simulink model "rotpentemplate_cleanedup"  (R2023a)
settings: Solver=VariableStepDiscrete  StartTime=0.0  StopTime=120  RelTol=1e-3  EnableMultiTasking=on
values from neighbouring files (symbols this model uses):
  adingain = [adingain 1 1 1 1 1]    [hwinit.m]    (also in theta2_bottomswing.mat = [1.276 1.276 1 1 1 1 1])
  adinoffs = [adinoffs 0 0 0 0 0]    [hwinit.m]    (also in theta2_bottomswing.mat = [-3.773 -1.223 0 0 0 0 0])
  daoutgain = 1*[-6]    [hwinit.m]    (also in theta2_bottomswing.mat = -6)
  daoutoffs = [0.00]    [hwinit.m]    (also in theta2_bottomswing.mat = 0)
  h = 0.01    [hwinit.m]    (also in mpc_controller.m = zeros(dim.nx+dim.nu, 1); theta2_bottomswing.mat = 0.05)
  K_lqr = [K_lqr, 0, 0]    [mpc_controller.m]
  sys_dis = c2d(sys_ct, h)    [mpc_controller.m]
undefined symbols (not defined in the file or in its folder): DiscIntNeverNeededParam, Discrete, Time
libraries: simulink x3, ctrlSharedLib x1
settings Model: Creator=rbabuska  LastModifiedBy=ellyb
settings SolverCC: AlgebraicLoopSolver=TrustRegion
settings DataIOCC: LimitDataPoints=on  SaveFormat=Array  ReturnWorkspaceOutputs=off  SignalLoggingName=sigsOut
settings OptimizationCC: BooleanDataType=off  ExpressionDepthLimit=2147483647  InitFltsAndDblsToZero=on  LifeSpan=inf
settings DebuggingCC: SaveWithParameterizedLinksMsg=none  SignalResolutionControl=TryResolveAllWithWarning  MultiTaskDSMMsg=warning  MultiTaskCondExecSysMsg=none  UnconnectedInputMsg=warning  UnconnectedOutputMsg=warning  UnconnectedLineMsg=warning  AllowSymbolicDim=off  StateNameClashWarn=warning  SFUnexpectedBacktrackingDiag=warning  SFNoUnconditionalDefaultTransitionDiag=warning  SFExecutionAtInitializationDiag=none  ArithmeticOperatorsInVariantConditions=warning
settings HardwareCC: ProdBitPerPointer=32  ProdBitPerSizeT=32  ProdBitPerPtrDiffT=32  ProdLargestAtomicFloat=None  ProdIntDivRoundTo=Undefined  ProdEndianess=Unspecified  ProdWordSize=32  ProdHWDeviceType=32-bit Generic  TargetUnknown=on
settings ModelReferenceCC: EnableRefExpFcnMdlSchedulingChecks=on  PropagateSignalLabelsOutOfModel=off
settings SFSimCC: SimUseLocalCustomCode=off  CustomCodeUndefinedFunction=UseInterfaceOnly
settings RTWCC: RTWUseLocalCustomCode=off  DLArmComputeVersion=19.05
settings CodeAppCC: StateflowObjectComments=on
settings GRTTargetCC: TargetFcnLib=ansi_tfl_tmw.mat  TargetLangStandard=C89/C90 (ANSI)  CombineOutputUpdateFcns=off  GRTInterface=on
settings ConfigComp: CovMetricSettings=dw  CovSaveCumulativeToWorkspaceVar=on  CovSaveSingleToWorkspaceVar=on  CovExternalEMLEnable=off

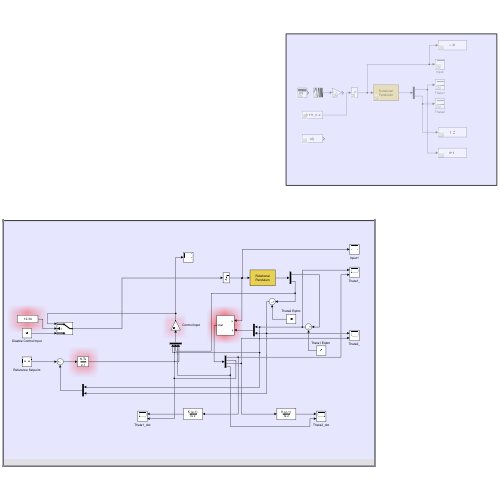
[thumbnail: Simulink's stored preview of the top-level diagram]
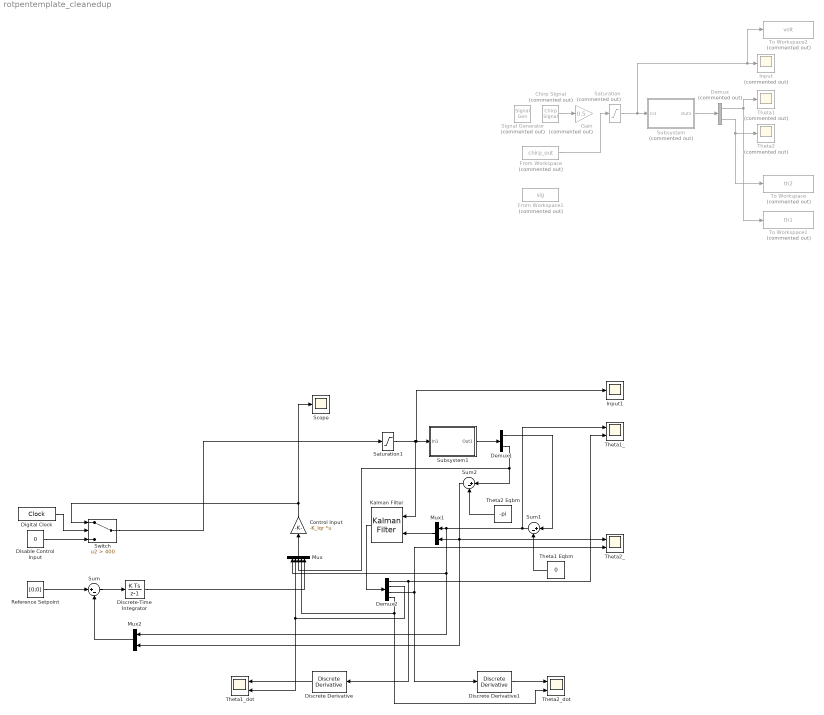
== system rotpentemplate_cleanedup ==
  Chirp Signal : simulink/Sources/Chirp Signal  Commented=on  f1=2  T=45  f2=6
  Control Input : Gain  Gain=-K_lqr  Multiplication=Matrix(K*u)
  Demux : Demux  Commented=on  Outputs=2
  Demux1 : Demux  Outputs=2
  Demux2 : Demux
  Digital Clock : DigitalClock  SampleTime=h
  Disable Control Input : Constant  Value=0  SampleTime=-1
  Discrete Derivative : simulink/Discrete/Discrete Derivative  gainval=1.0  ICPrevScaledInput=0.0  OutMin=[]  OutMax=[]  OutDataType=fixdt(1, 16)  OutScaling=2^-10  DoSatur=off
  Discrete Derivative1 : simulink/Discrete/Discrete Derivative  gainval=1.0  ICPrevScaledInput=0.0  OutMin=[]  OutMax=[]  OutDataType=fixdt(1, 16)  OutScaling=2^-10  DoSatur=off
  Discrete-Time Integrator : DiscreteIntegrator  SampleTime=h  ICPrevOutput=DiscIntNeverNeededParam  ICPrevScaledInput=DiscIntNeverNeededParam
  From Workspace : FromWorkspace  Commented=on  VariableName=chirp_out  SampleTime=h
  From Workspace1 : FromWorkspace  Commented=on  VariableName=sig  SampleTime=h
  Gain : Gain  Commented=on  Gain=0.5
  Input : Scope  Commented=on
  Input1 : Scope
  Kalman Filter : ctrlSharedLib/Kalman Filter  TimeDomain=Discrete-Time  UseCurrentEstimator=on  ModelSource=Individual A, B, C, D matrices  ModelSourceVariable=ss(0.95,1,1,0,1)  A=sys_dis.A  B=sys_dis.B  C=sys_dis.C  D=sys_dis.D  NumberOfStates=1  NumberOfInputs=1  NumberOfOutputs=1  InitialEstimateSource=Dialog  X0=0  P0=10  UseK=off  UseGH=off  NumberOfProcessNoiseInputs=1  G=1  TimeInvariantG=on  H=0  TimeInvariantH=on  Q=diag([0.1^2 0.1^2 0.01^2 0.001^2])  TimeInvariantQ=on  R=diag([0.01^2 0.05^2])  TimeInvariantR=on  N=0  TimeInvariantN=on  AddInputPort=on  AddEnablePort=off  OutputEstimatedY=off  OutputP=off  Ts=-1
  Mux : Mux  Inputs=5
  Mux1 : Mux  Inputs=2
  Mux2 : Mux  Inputs=2
  Reference Setpoint : Constant  Value=[0;0]  SampleTime=-1
  Saturation : Saturate  Commented=on  UpperLimit=1  LowerLimit=-1
  Saturation1 : Saturate  UpperLimit=1  LowerLimit=-1
  Scope : Scope
  Signal Generator : SignalGenerator  Commented=on  Amplitude=0.3*1
  Subsystem : Subsystem  Commented=on
      mask Display: disp('Rotational\nPendulum')
  Subsystem1 : Subsystem
      mask Display: disp('Rotational\nPendulum')
  Sum : Sum  Inputs=|+-
  Sum1 : Sum  Inputs=|+-
  Sum2 : Sum  Inputs=|+-
  Switch : Switch  Criteria=u2 > Threshold  Threshold=400  SaturateOnIntegerOverflow=off  InputSameDT=off
  Theta1 : Scope  Commented=on
  "Theta1 Eqbm " : Constant  Value=0  SampleTime=-1
  Theta1_ : Scope  NumInputPorts=2
  Theta1_dot : Scope  NumInputPorts=2
  Theta2 : Scope  Commented=on
  Theta2 Eqbm : Constant  Value=-pi  SampleTime=-1
  Theta2_ : Scope  NumInputPorts=2
  Theta2_dot : Scope  NumInputPorts=2
  To Workspace : ToWorkspace  Commented=on  VariableName=th2  SaveFormat=Timeseries  SampleTime=-1
  To Workspace1 : ToWorkspace  Commented=on  VariableName=th1  SaveFormat=Timeseries  SampleTime=-1
  To Workspace2 : ToWorkspace  Commented=on  VariableName=volt  SaveFormat=Timeseries  SampleTime=-1
  wires:
  Saturation/1 -> Subsystem/1(In1), To Workspace2/1, Input/1
  Subsystem/1(Out1) -> Demux/1
  Demux/1 -> To Workspace1/1, Theta1/1
  Demux/2 -> To Workspace/1, Theta2/1
  Chirp Signal/1 -> Gain/1
  From Workspace/1 -> Saturation/1
  Demux1/1 -> Sum1/1
  Demux1/2 -> Sum2/1, Mux/3
  Subsystem1/1(Out1) -> Demux1/1
  Saturation1/1 -> Subsystem1/1(In1), Input1/1, Kalman Filter/1
  Kalman Filter/1 -> Demux2/1
  Demux2/3 -> Theta2_/2, Discrete Derivative1/1
  Mux/1 -> Control Input/1
  Demux2/2 -> Theta1_dot/2, Mux/2
  Demux2/1 -> Theta1_/2, Discrete Derivative/1
  Demux2/4 -> Theta2_dot/2, Mux/4
  "Theta1 Eqbm "/1 -> Sum1/2
  Mux1/1 -> Kalman Filter/2
  Discrete Derivative1/1 -> Theta2_dot/1
  Discrete Derivative/1 -> Theta1_dot/1
  Theta2 Eqbm/1 -> Sum2/2
  Sum2/1 -> Mux1/2, Mux2/2, Theta2_/1
  Sum1/1 -> Mux2/1, Mux/1, Mux1/1, Theta1_/1
  Switch/1 -> Saturation1/1
  Control Input/1 -> Scope/1, Switch/1
  Digital Clock/1 -> Switch/2
  Disable Control Input/1 -> Switch/3
  Sum/1 -> Discrete-Time Integrator/1
  Mux2/1 -> Sum/2
  Reference Setpoint/1 -> Sum/1
  Discrete-Time Integrator/1 -> Mux/5

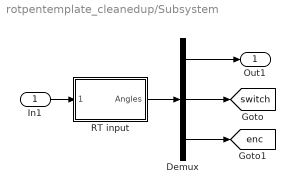
== system rotpentemplate_cleanedup/Subsystem ==
  In1 : Inport
  Demux : Demux  Outputs=[2 4 1]
  RT input : Subsystem  mask{Ts=h, channels=[6 7]}
      mask prompts: Ts "Sample time [s]:"; channels "Channels to read (e.g., [6 7])"
      mask init:
      | hwinit;
      | 
      | % initialize FPGA
      | fugihandle = fugiboard('Open', 'Pendulum1');
      | fugihandle.WatchdogTimeout = 0.5;
      | fugiboard('SetParams', fugihandle);
      | fugiboard('Write', fugihandle, 0, 0, 0, 0);  % dummy write to sync interface board
      | fugiboard('Write', fugihandle, 5, 1, 0, 0);  % reset position, activate relay
      | data = fugiboard('Read', fugihandle);        % get version info from FPGA
      | % model = bitshift(data(1), -5); 
      | % version = bitand(data(1), 31);
      | % disp(sprintf('FPGA setup %d, version %d', model, version)); % for the B&P it should say 1 1, or else there is a problem
      | fugiboard('Write', fugihandle, 0, 1, 0, 0);  % end reset
      | pause(0.1);                         % give relay some time to respond
      mask Display: disp('Rotational\nPendulum')
  Out1 : Outport
  tag scope: enc=global, switch=global
  wires:
  RT input/1(Angles) -> Demux/1
  Demux/1 -> Out1/1
  Demux/2 -> [switch]
  Demux/3 -> [enc]
  In1/1 -> RT input/1(Motors)

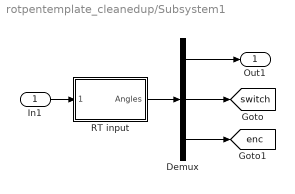
== system rotpentemplate_cleanedup/Subsystem1 ==
  In1 : Inport
  Demux : Demux  Outputs=[2 4 1]
  RT input : Subsystem  mask{Ts=h, channels=[6 7]}
      mask prompts: Ts "Sample time [s]:"; channels "Channels to read (e.g., [6 7])"
      mask init: same as rotpentemplate_cleanedup/Subsystem/RT input
      mask Display: disp('Rotational\nPendulum')
  Out1 : Outport
  tag scope: enc=global, switch=global
  wires:
  RT input/1(Angles) -> Demux/1
  Demux/1 -> Out1/1
  Demux/2 -> [switch]
  Demux/3 -> [enc]
  In1/1 -> RT input/1(Motors)

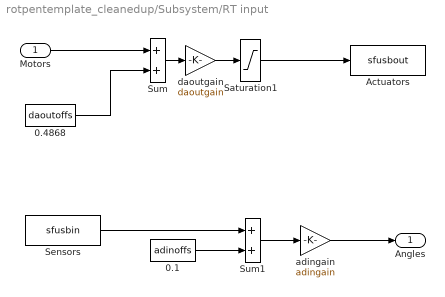
== system rotpentemplate_cleanedup/Subsystem/RT input ==
  Motors : Inport
  0.1 : Constant  Value=adinoffs
  0.4868 : Constant  Value=daoutoffs
  Actuators : S-Function  FunctionName=sfusbout  Parameters=Ts, fugihandle  SFunctionDeploymentMode=off  EnableBusSupport=off
  Saturation1 : Saturate  UpperLimit=10  LowerLimit=-10
  Sensors : S-Function  FunctionName=sfusbin  Parameters=Ts, fugihandle, channels  SFunctionDeploymentMode=off  EnableBusSupport=off
  Sum : Sum  InputSameDT=on  SaturateOnIntegerOverflow=on  OutDataTypeStr=Inherit: Same as first input
  Sum1 : Sum  InputSameDT=on  SaturateOnIntegerOverflow=on  OutDataTypeStr=Inherit: Same as first input
  adingain : Gain  Gain=adingain  SaturateOnIntegerOverflow=on  OutDataTypeStr=Inherit: Same as input  ParamDataTypeStr=Inherit: Same as input
  daoutgain : Gain  Gain=daoutgain  SaturateOnIntegerOverflow=on  OutDataTypeStr=Inherit: Same as input  ParamDataTypeStr=Inherit: Same as input
  Angles : Outport
  wires:
  Sum/1 -> daoutgain/1
  0.4868/1 -> Sum/2
  Motors/1 -> Sum/1
  Sum1/1 -> adingain/1
  0.1/1 -> Sum1/2
  adingain/1 -> Angles/1
  Saturation1/1 -> Actuators/1
  daoutgain/1 -> Saturation1/1
  Sensors/1 -> Sum1/1

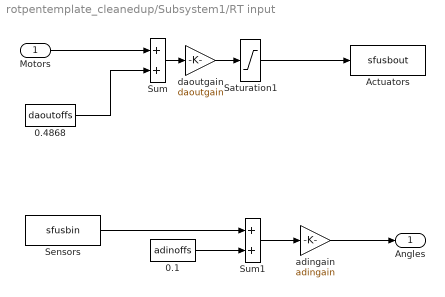
== system rotpentemplate_cleanedup/Subsystem1/RT input ==
  Motors : Inport
  0.1 : Constant  Value=adinoffs
  0.4868 : Constant  Value=daoutoffs
  Actuators : S-Function  FunctionName=sfusbout  Parameters=Ts, fugihandle  SFunctionDeploymentMode=off  EnableBusSupport=off
  Saturation1 : Saturate  UpperLimit=10  LowerLimit=-10
  Sensors : S-Function  FunctionName=sfusbin  Parameters=Ts, fugihandle, channels  SFunctionDeploymentMode=off  EnableBusSupport=off
  Sum : Sum  InputSameDT=on  SaturateOnIntegerOverflow=on  OutDataTypeStr=Inherit: Same as first input
  Sum1 : Sum  InputSameDT=on  SaturateOnIntegerOverflow=on  OutDataTypeStr=Inherit: Same as first input
  adingain : Gain  Gain=adingain  SaturateOnIntegerOverflow=on  OutDataTypeStr=Inherit: Same as input  ParamDataTypeStr=Inherit: Same as input
  daoutgain : Gain  Gain=daoutgain  SaturateOnIntegerOverflow=on  OutDataTypeStr=Inherit: Same as input  ParamDataTypeStr=Inherit: Same as input
  Angles : Outport
  wires:
  Sum/1 -> daoutgain/1
  0.4868/1 -> Sum/2
  Motors/1 -> Sum/1
  Sum1/1 -> adingain/1
  0.1/1 -> Sum1/2
  adingain/1 -> Angles/1
  Saturation1/1 -> Actuators/1
  daoutgain/1 -> Saturation1/1
  Sensors/1 -> Sum1/1
